simulink model "buoyancy_simulation"  (R2021a)
settings: Solver=ode45  StartTime=0.0  StopTime=180  MaxStep=2.0  RelTol=1e-3
values from neighbouring files (symbols this model uses):
  Cd_bottom = 1    [main_simulation.m]
  Cd_top = 1.28    [main_simulation.m]
  densityProfile = 999    [main_simulation.m]
  depth_CTD = depth_CTD(1:index)    [main_simulation.m]
  g = 9.81    [main_simulation.m]
  integralTreshold = 2    [main_simulation.m]
  Kd = 0.1    [main_simulation.m]
  Ki = 0.001    [main_simulation.m]
  Kp = 0.026    [main_simulation.m]
  offsetSensor = 0    [main_simulation.m]
  sampleTime = 0.5    [main_simulation.m]
  step_depth1 = 10    [main_simulation.m]
  step_depth2 = 5    [main_simulation.m]
  stepTime = 180    [main_simulation.m]
  useCTDprofile = true    [main_simulation.m]
  V_max = V_vehicle + V_outerLid + V_led - V_pistonBlock - V_sensor    [calc_preset_volume.m]
  v_piston_max = 2.44e-3    (= 0.00244)    [main_simulation.m]
undefined symbols (not defined in the file or in its folder): mass, param, rho, sysc
libraries: pid_lib x1
settings Model: Creator=haral  LastModifiedBy=haral
settings SolverCC: ZeroCrossAlgorithm=Adaptive
settings DebuggingCC: IgnoredZcDiagnostic=none

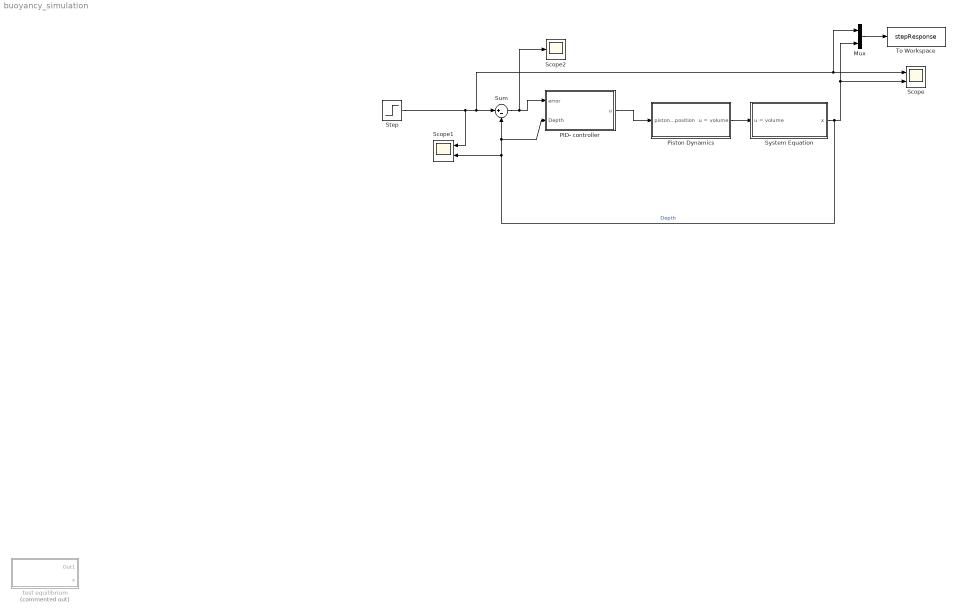
== system buoyancy_simulation ==
  Mux : Mux  Inputs=2
  PID- controller : Subsystem
  Piston Dynamics : Subsystem
  Scope : Scope  NumInputPorts=2
  Scope1 : Scope  NumInputPorts=2
  Scope2 : Scope
  Step : Step  Time=stepTime  Before=step_depth1  After=step_depth2  SampleTime=sampleTime
  Sum : Sum  Inputs=|+-
  System Equation : Subsystem
  To Workspace : ToWorkspace  VariableName=stepResponse  SaveFormat=Structure With Time  SampleTime=-1
  test equilibrium : Subsystem  Commented=on
  wires:
  Step/1 -> Scope1/1, Mux/1, Scope/1, Sum/1
  Sum/1 -> Scope2/1, PID- controller/1(error)
  PID- controller/1(u) -> Piston Dynamics/1(piston position)
  Piston Dynamics/1(u = volume) -> System Equation/1(u = volume)
  System Equation/1(x) -> Sum/2, PID- controller/2(Depth), Scope1/2, Mux/2, Scope/2  "Depth"
  Mux/1 -> To Workspace/1

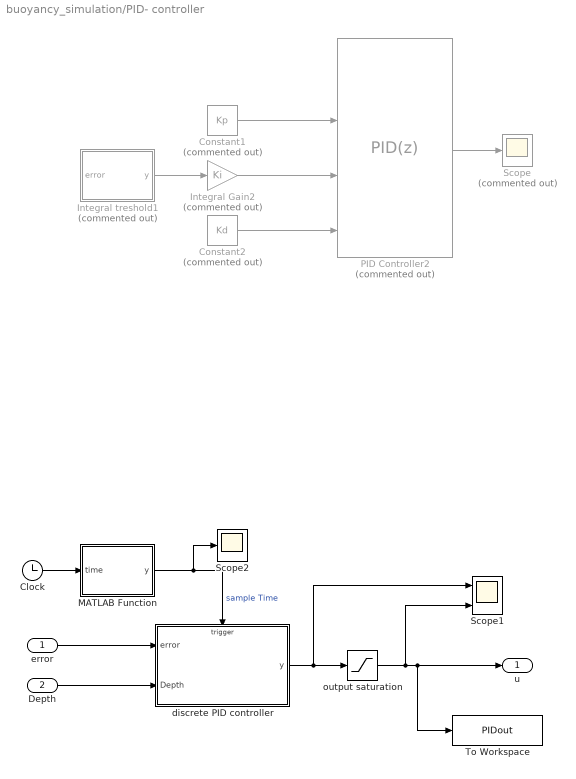
== system buoyancy_simulation/PID- controller ==
  error : Inport
  Depth : Inport  Port=2
  Clock : Clock
  Constant1 : Constant  Commented=on  Value=Kp
  Constant2 : Constant  Commented=on  Value=Kd
  Integral Gain2 : Gain  Commented=on  Gain=Ki
  Integral treshold1 : MATLAB Function  Commented=on  TreatAsAtomicUnit=on
  MATLAB Function : MATLAB Function  TreatAsAtomicUnit=on
  PID Controller2 : pid_lib/PID Controller  Commented=on  Controller=PID  Form=Parallel  TimeDomain=Discrete-time  UseExternalTs=off  SampleTime=0.5  IntegratorMethod=Forward Euler  FilterMethod=Forward Euler  ControllerParametersSource=external  P=Kp  I=Ki  D=Kd  UseFilter=off  N=72.1075704960884  TunerSelectOption=Transfer Function Based (PID Tuner App)  ZeroCross=off  InitialConditionSource=internal  InitialConditionForIntegrator=0  InitialConditionForFilter=0  DifferentiatorICPrevScaledInput=0  ExternalReset=none  TrackingMode=off  Kt=1  LimitOutput=on  SatLimitsSource=internal  UpperSaturationLimit=inf  LowerSaturationLimit=0  LinearizeAsGain=on  AntiWindupMode=none  Kb=1  POutMin=[]  POutMax=[]  IOutMin=[]  IOutMax=[]  DOutMin=[]  DOutMax=[]  NOutMin=[]  NOutMax=[]  SumOutMin=[]  SumOutMax=[]  SaturationOutMin=[]  SaturationOutMax=[]  PParamMin=[]  PParamMax=[]  IParamMin=[]  IParamMax=[]  DParamMin=[]  DParamMax=[]  NParamMin=[]  NParamMax=[]  KbParamMin=[]  KbParamMax=[]  KtParamMin=[]  KtParamMax=[]  KbOutMin=[]  KbOutMax=[]  KtOutMin=[]  KtOutMax=[]  IntegratorOutMin=[]  IntegratorOutMax=[]  FilterOutMin=[]  FilterOutMax=[]  SumI1OutMin=[]  SumI1OutMax=[]  SumI2OutMin=[]  SumI2OutMax=[]  SumI3OutMin=[]  SumI3OutMax=[]  SumI4OutMin=[]  SumI4OutMax=[]  SumDOutMin=[]  SumDOutMax=[]  DifferentiatorOutMin=[]  DifferentiatorOutMax=[]  FilterDiffOutCoefMin=[]  FilterDiffOutCoefMax=[]  ReciprocalOutMin=[]  ReciprocalOutMax=[]  SumDenOutMin=[]  SumDenOutMax=[]  SumNumOutMin=[]  SumNumOutMax=[]  DivideOutMin=[]  DivideOutMax=[]  UdiffTsProdOutMin=[]  UdiffTsProdOutMax=[]  NTsProdOutMin=[]  NTsProdOutMax=[]  UintegralTsProdOutMin=[]  UintegralTsProdOutMax=[]  UngainTsProdOutMin=[]  UngainTsProdOutMax=[]  IntegratorContinuousStateAttributes=''  IntegratorStateMustResolveToSignalObject=off  IntegratorRTWStateStorageClass=Auto  FilterContinuousStateAttributes=''  FilterStateMustResolveToSignalObject=off  FilterRTWStateStorageClass=Auto  ParallelPVariant=ExternalParameters  IdealPVariant=Disabled  IVariant=ExternalParameters  DVariant=ExternalParameters  IntegratorVariant=Discrete  SatVariant=Enabled  AWVariant=Passthrough  PCopyVariant=Disabled  TRVariant=Disabled  FdbkBlocksVariant=Forward  IdealPFdbkVariant=Disabled  SatFdbkVariant=Disabled  DerivativeFilterVariant=Differentiator  NVariant=Passthrough  NCopyVariant=Disabled_SignalSpec  FilterICVariant=InternalICsDifferentiator  IntegratorICVariant=InternalICs  ExternalResetVariant=Disabled  TRSumVariant=Passthrough  SumFdbkVariant=Disabled  SumVariant=Sum_PID  TsampFilterVariant=InternalTs  TsampNgainVariant=Passthrough  TsampIntegralVariant=Passthrough  ExternalSaturationOutDataTypeStr=Inherit: Same as second input
  Scope : Scope  Commented=on
  Scope1 : Scope  NumInputPorts=2
  Scope2 : Scope
  To Workspace : ToWorkspace  VariableName=PIDout  SaveFormat=Structure With Time  SampleTime=-1
  "discrete PID controller " : Subsystem  TreatAsAtomicUnit=on
  output saturation : Saturate  UpperLimit=param.h_piston  LowerLimit=0
  u : Outport
  wires:
  Integral treshold1/1(y) -> Integral Gain2/1
  Constant2/1 -> PID Controller2/4
  Integral Gain2/1 -> PID Controller2/3
  Constant1/1 -> PID Controller2/2
  error/1 -> "discrete PID controller "/1(error)
  "discrete PID controller "/1(y) -> Scope1/1, output saturation/1
  output saturation/1 -> To Workspace/1, u/1, Scope1/2
  MATLAB Function/1(y) -> Scope2/1, "discrete PID controller "/Trigger  "sample Time"
  Clock/1 -> MATLAB Function/1(time)
  PID Controller2/1 -> Scope/1
  Depth/1 -> "discrete PID controller "/2(Depth)

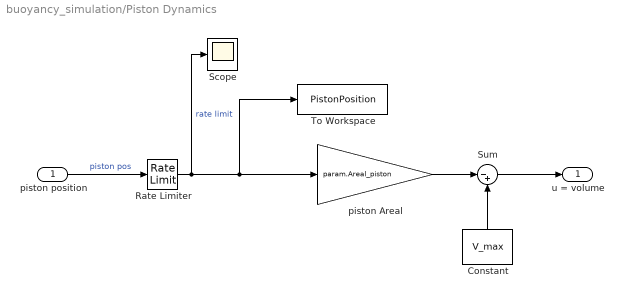
== system buoyancy_simulation/Piston Dynamics ==
  piston position : Inport
  Constant : Constant  Value=V_max
  Rate Limiter : RateLimiter  RisingSlewLimit=v_piston_max  FallingSlewLimit=-v_piston_max  SampleTimeMode=inherited
  Scope : Scope
  Sum : Sum  Inputs=|-+
  To Workspace : ToWorkspace  VariableName=PistonPosition  SaveFormat=Structure With Time  SampleTime=-1
  piston Areal : Gain  Gain=param.Areal_piston
  u = volume : Outport
  wires:
  Rate Limiter/1 -> Scope/1, To Workspace/1, piston Areal/1  "rate limit"
  piston position/1 -> Rate Limiter/1  "piston pos"
  Constant/1 -> Sum/2
  piston Areal/1 -> Sum/1
  Sum/1 -> u = volume/1

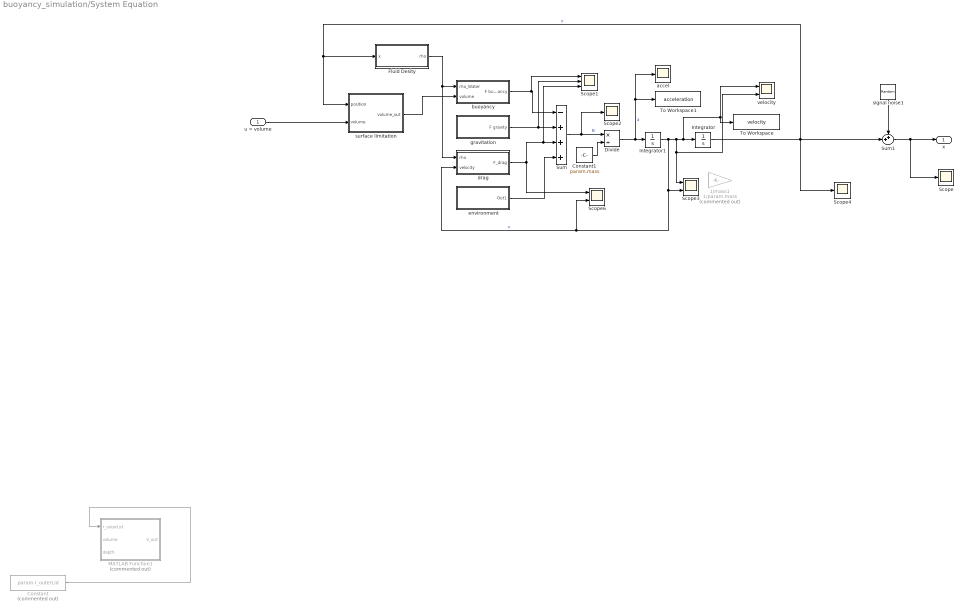
== system buoyancy_simulation/System Equation ==
  u = volume : Inport
  1/mass1 : Gain  Commented=on  Gain=1/param.mass
  Constant : Constant  Commented=on  Value=param.r_outerLid
  Constant1 : Constant  Value=param.mass
  Divide : Product  Inputs=*/
  Fluid Desity : Subsystem
  Integrator : Integrator
  Integrator1 : Integrator
  MATLAB Function1 : MATLAB Function  Commented=on  TreatAsAtomicUnit=on
  Scope : Scope
  Scope1 : Scope  NumInputPorts=3
  Scope2 : Scope
  Scope3 : Scope  NumInputPorts=2
  Scope4 : Scope
  Scope6 : Scope  NumInputPorts=2
  Sum : Sum  Inputs=-+++
  Sum1 : Sum  Inputs=++|
  To Workspace : ToWorkspace  VariableName=velocity  SaveFormat=Structure With Time  SampleTime=-1
  To Workspace1 : ToWorkspace  VariableName=acceleration  SaveFormat=Structure With Time  SampleTime=-1
  accel : Scope
  buoyancy : Subsystem
  drag : Subsystem
  environment : Subsystem
  gravitation : Subsystem
  signal noise1 : RandomNumber  Variance=0.0001  SampleTime=0.5
  surface limitation : MATLAB Function  TreatAsAtomicUnit=on
  velocity : Scope  NumInputPorts=2
  x : Outport
  wires:
  Divide/1 -> accel/1, To Workspace1/1, Integrator1/1  "a"
  Integrator1/1 -> Scope6/2, drag/2(velocity), Scope3/2, velocity/2, Scope3/1, velocity/1, To Workspace/1, Integrator/1  "v"
  buoyancy/1(F buoyancy) -> Scope1/1, Sum/1
  gravitation/1(F gravity) -> Scope1/2, Sum/2
  drag/1(F_drag) -> Scope1/3, Sum/3, Scope6/1
  environment/1(Out1) -> Sum/4
  Fluid Desity/1(rho) -> drag/1(rho), buoyancy/1(rho_Water)
  Sum/1 -> Divide/1, Scope2/1  "N"
  u = volume/1 -> surface limitation/2(volume)
  Integrator/1 -> Sum1/2, surface limitation/1(position), Fluid Desity/1(x), Scope4/1  "x"
  Constant/1 -> MATLAB Function1/1(r_outerLid)
  surface limitation/1(volume_out) -> buoyancy/2(volume)
  signal noise1/1 -> Sum1/1
  Sum1/1 -> Scope/1, x/1
  Constant1/1 -> Divide/2

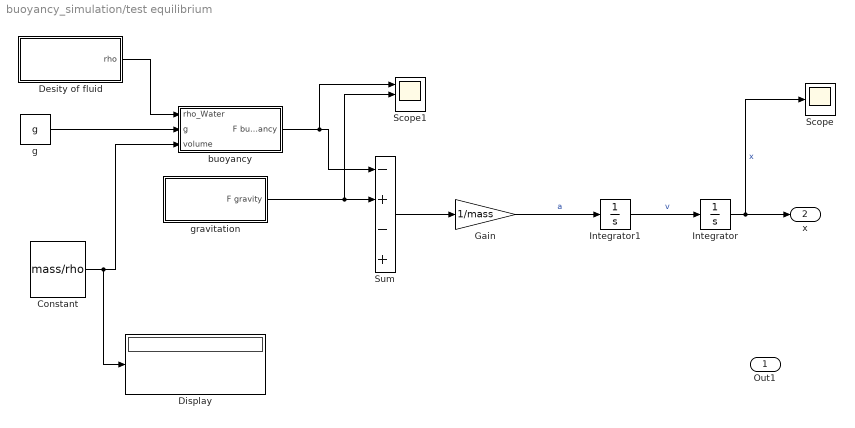
== system buoyancy_simulation/test equilibrium ==
  Constant : Constant  Value=mass/rho
  Desity of fluid : Subsystem
  Display : Display
  Gain : Gain  Gain=1/mass
  Integrator : Integrator
  Integrator1 : Integrator
  Scope : Scope
  Scope1 : Scope  NumInputPorts=3
  Sum : Sum  Inputs=-+-+
  buoyancy : Subsystem
  g : Constant  Value=g
  gravitation : Subsystem
  Out1 : Outport
  x : Outport  Port=2
  wires:
  Constant/1 -> Display/1, buoyancy/3(volume)
  g/1 -> buoyancy/2(g)
  buoyancy/1(F buoyancy) -> Scope1/1, Sum/1
  Gain/1 -> Integrator1/1  "a"
  Integrator/1 -> Scope/1, x/1  "x"
  Desity of fluid/1(rho) -> buoyancy/1(rho_Water)
  Integrator1/1 -> Integrator/1  "v"
  Sum/1 -> Gain/1
  gravitation/1(F gravity) -> Scope1/2, Sum/2

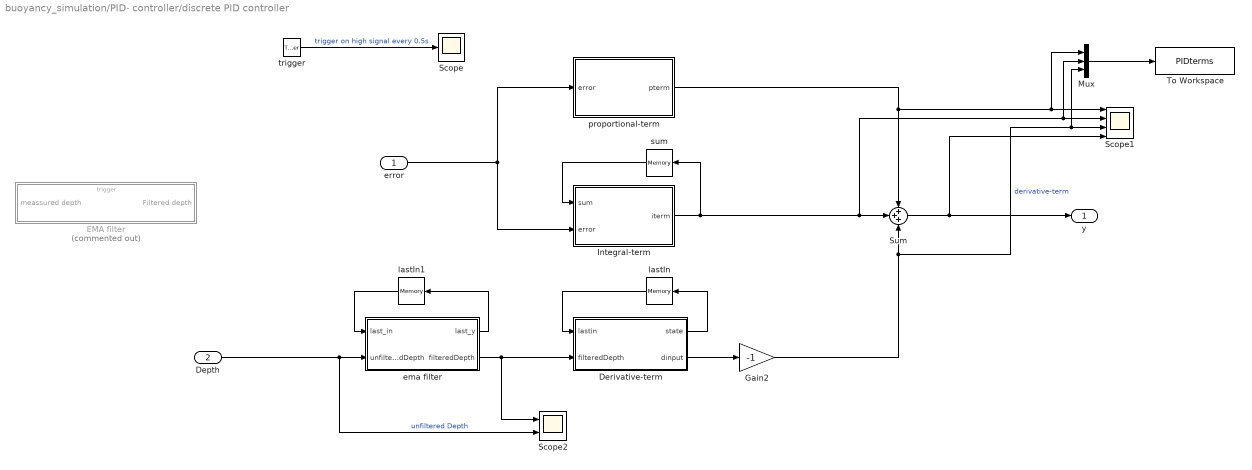
== system buoyancy_simulation/PID- controller/discrete PID controller  ==
  error : Inport
  Depth : Inport  Port=2
  trigger : TriggerPort  VariantControl=(inherit)  ShowOutputPort=on  SampleTimeType=periodic  SampleTime=sampleTime
  Derivative-term : MATLAB Function  TreatAsAtomicUnit=on
  EMA filter : Subsystem  Commented=on
  Gain2 : Gain  Gain=-1
  Integral-term : MATLAB Function  TreatAsAtomicUnit=on
  Mux : Mux  Inputs=3
  Scope : Scope
  Scope1 : Scope  NumInputPorts=4
  Scope2 : Scope  NumInputPorts=2
  Sum : Sum  Inputs=+++
  To Workspace : ToWorkspace  VariableName=PIDterms  SaveFormat=Structure With Time  SampleTime=-1
  ema filter : MATLAB Function  TreatAsAtomicUnit=on
  lastIn : Memory  InheritSampleTime=on
  lastIn1 : Memory  InheritSampleTime=on
  proportional-term : MATLAB Function  TreatAsAtomicUnit=on
  sum : Memory  InheritSampleTime=on
  y : Outport
  wires:
  Integral-term/1(iterm) -> sum/1, Mux/2, Scope1/2, Sum/2
  sum/1 -> Integral-term/1(sum)
  error/1 -> Integral-term/2(error), proportional-term/1(error)
  Depth/1 -> Scope2/2, ema filter/2(unfilteredDepth)  "unfiltered Depth"
  Derivative-term/1(state) -> lastIn/1
  lastIn/1 -> Derivative-term/1(lastin)
  Derivative-term/2(dinput) -> Gain2/1
  Gain2/1 -> Mux/3, Scope1/3, Sum/3  "derivative-term"
  proportional-term/1(pterm) -> Sum/1, Mux/1, Scope1/1
  Sum/1 -> Scope1/4, y/1
  trigger/1 -> Scope/1  "trigger on high signal every 0.5s"
  Mux/1 -> To Workspace/1
  lastIn1/1 -> ema filter/1(last_in)
  ema filter/1(last_y) -> lastIn1/1
  ema filter/2(filteredDepth) -> Scope2/1, Derivative-term/2(filteredDepth)

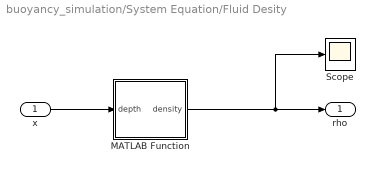
== system buoyancy_simulation/System Equation/Fluid Desity ==
  x : Inport
  MATLAB Function : MATLAB Function  TreatAsAtomicUnit=on
  Scope : Scope
  rho : Outport
  wires:
  MATLAB Function/1(density) -> rho/1, Scope/1
  x/1 -> MATLAB Function/1(depth)

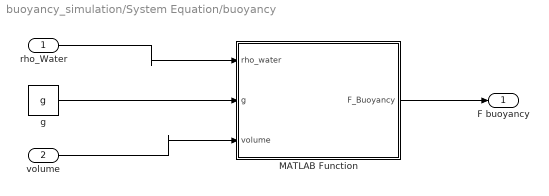
== system buoyancy_simulation/System Equation/buoyancy ==
  rho_Water : Inport
  volume : Inport  Port=2
  MATLAB Function : MATLAB Function  TreatAsAtomicUnit=on
  g : Constant  Value=g
  F buoyancy : Outport
  wires:
  rho_Water/1 -> MATLAB Function/1(rho_water)
  g/1 -> MATLAB Function/2(g)
  volume/1 -> MATLAB Function/3(volume)
  MATLAB Function/1(F_Buoyancy) -> F buoyancy/1

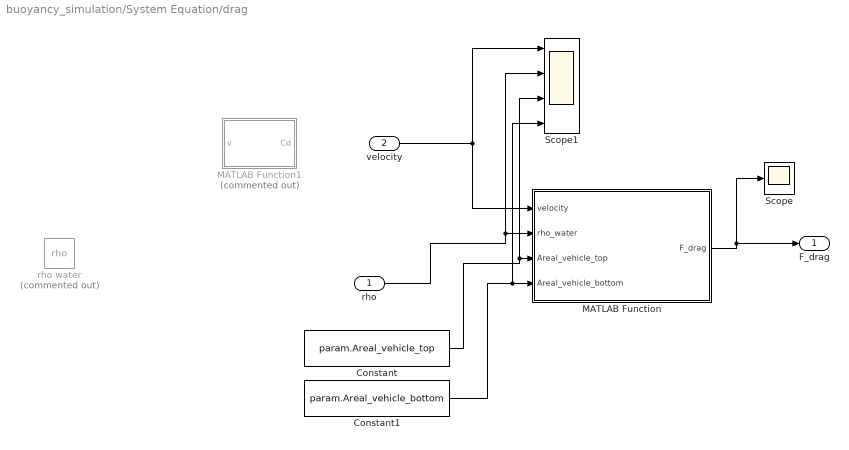
== system buoyancy_simulation/System Equation/drag ==
  rho : Inport
  velocity : Inport  Port=2
  Constant : Constant  Value=param.Areal_vehicle_top
  Constant1 : Constant  Value=param.Areal_vehicle_bottom
  MATLAB Function : MATLAB Function  TreatAsAtomicUnit=on
  MATLAB Function1 : MATLAB Function  Commented=on  TreatAsAtomicUnit=on
  Scope : Scope
  Scope1 : Scope  NumInputPorts=4
  rho water : Constant  Commented=on  Value=rho
  F_drag : Outport
  wires:
  velocity/1 -> Scope1/1, MATLAB Function/1(velocity)
  Constant/1 -> Scope1/3, MATLAB Function/3(Areal_vehicle_top)
  MATLAB Function/1(F_drag) -> Scope/1, F_drag/1
  rho/1 -> Scope1/2, MATLAB Function/2(rho_water)
  Constant1/1 -> Scope1/4, MATLAB Function/4(Areal_vehicle_bottom)

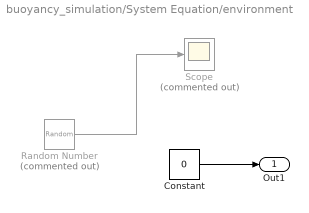
== system buoyancy_simulation/System Equation/environment ==
  Constant : Constant  Value=0
  Random Number : RandomNumber  Commented=on  Variance=0.001  SampleTime=0.1
  Scope : Scope  Commented=on
  Out1 : Outport
  wires:
  Random Number/1 -> Scope/1
  Constant/1 -> Out1/1

== system buoyancy_simulation/System Equation/gravitation ==
  Constant : Constant  Value=param.mass
  Gain : Gain  Gain=g
  F gravity : Outport
  wires:
  Gain/1 -> F gravity/1
  Constant/1 -> Gain/1

== system buoyancy_simulation/test equilibrium/Desity of fluid ==
  Constant : Constant  Value=1000
  rho : Outport
  wires:
  Constant/1 -> rho/1

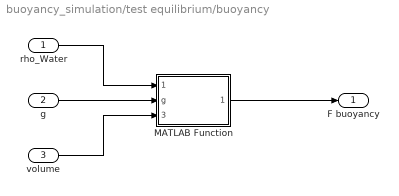
== system buoyancy_simulation/test equilibrium/buoyancy ==
  rho_Water : Inport
  g : Inport  Port=2
  volume : Inport  Port=3
  MATLAB Function : MATLAB Function  TreatAsAtomicUnit=on
  F buoyancy : Outport
  wires:
  rho_Water/1 -> MATLAB Function/1(rho_water)
  g/1 -> MATLAB Function/2(g)
  volume/1 -> MATLAB Function/3(volume)
  MATLAB Function/1(F_Buoyancy) -> F buoyancy/1

== system buoyancy_simulation/test equilibrium/gravitation ==
  Constant : Constant  Value=mass
  Gain : Gain  Gain=g
  F gravity : Outport
  wires:
  Gain/1 -> F gravity/1
  Constant/1 -> Gain/1

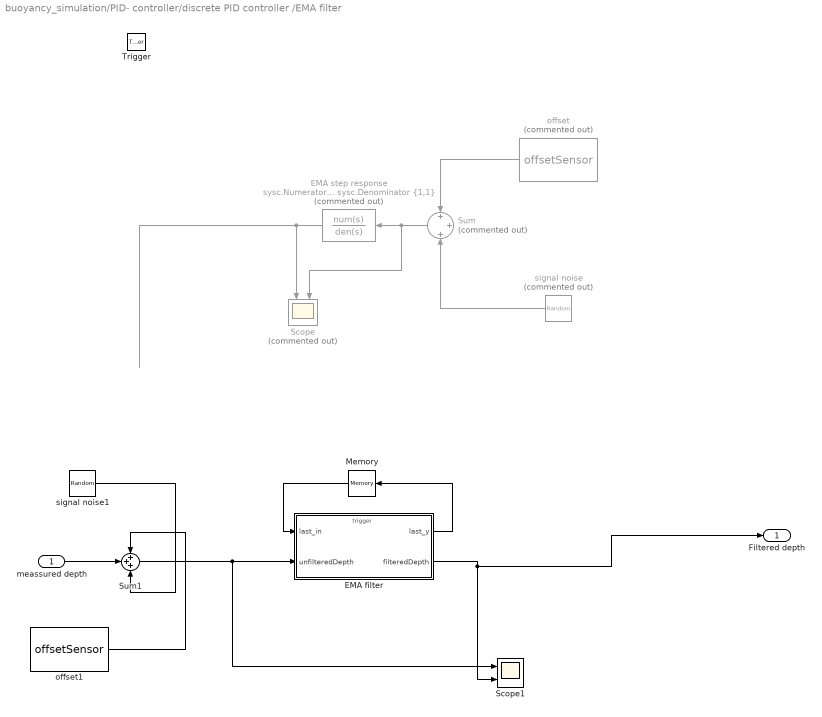
== system buoyancy_simulation/PID- controller/discrete PID controller /EMA filter ==
  meassured depth : Inport
  Trigger : TriggerPort  VariantControl=(inherit)  PortDimensions=1
  EMA filter : MATLAB Function  TreatAsAtomicUnit=on
  EMA step response : TransferFcn  Commented=on  Numerator=sysc.Numerator{1,1}  Denominator=sysc.Denominator {1,1}
  Memory : Memory  InheritSampleTime=on
  Scope : Scope  Commented=on  NumInputPorts=2
  Scope1 : Scope  NumInputPorts=2
  Sum : Sum  Commented=on  Inputs=+|+|+
  Sum1 : Sum  Inputs=+++
  offset : Constant  Commented=on  Value=offsetSensor
  offset1 : Constant  Value=offsetSensor
  signal noise : RandomNumber  Commented=on  Variance=0.0001  SampleTime=0.5
  signal noise1 : RandomNumber  Variance=0.0001  SampleTime=0.5
  Filtered depth : Outport
  wires:
  signal noise/1 -> Sum/3
  ? -> Sum/2
  offset/1 -> Sum/1
  Sum/1 -> Scope/2, EMA step response/1
  EMA step response/1 -> Scope/1
  EMA filter/1(last_y) -> Memory/1
  Memory/1 -> EMA filter/1(last_in)
  EMA filter/2(filteredDepth) -> Scope1/2, Filtered depth/1
  Sum1/1 -> EMA filter/2(unfilteredDepth), Scope1/1
  offset1/1 -> Sum1/1
  signal noise1/1 -> Sum1/3
  meassured depth/1 -> Sum1/2

== matlab function buoyancy_simulation/PID- controller/discrete PID controller /proportional-term ==
  settings: sampleTime=sampleTime
  data: error input; pterm output; Kp parameter
function pterm = fcn(error, Kp)

pterm = Kp*error;
end

== matlab function buoyancy_simulation/System Equation/surface limitation ==
  data: position input; volume input; volume_out output
function volume_out = fcn(position,volume)

if position <= 0
    volume_out = volume - pi*0.025^2*abs(position);
else
    volume_out = volume; 
end

== matlab function buoyancy_simulation/PID- controller/discrete PID controller /ema filter ==
  settings: sampleTime=sampleTime
  data: last_y output; last_in input; unfilteredDepth input; filteredDepth output; alpha parameter
function [last_y,filteredDepth ] = fcn(last_in, unfilteredDepth, alpha)

filteredDepth  =(alpha*unfilteredDepth) + ((1-alpha)*last_in);

%store variable for next calculation
last_y = filteredDepth;
end

== matlab function buoyancy_simulation/System Equation/drag/MATLAB Function1 ==
  data: v input; Cd output
function Cd = fcn(v)
%% not ideal lol
Cd = 0.130/((0.13/2)*(pi/4)*0.13^2*v^2);
end

== matlab function buoyancy_simulation/PID- controller/discrete PID controller /EMA filter/EMA filter ==
  settings: updateMethod=DISCRETE  sampleTime=sampleTime
  data: last_in input; unfilteredDepth input; last_y output; filteredDepth output; alpha parameter
  events: trigger input RISING_EDGE_EVENT
function [last_y,filteredDepth ] = fcn(last_in, unfilteredDepth, alpha)

filteredDepth  =(alpha*unfilteredDepth) + ((1-alpha)*last_in);

%store variable for next calculation
last_y = filteredDepth;
end

== matlab function buoyancy_simulation/System Equation/drag/MATLAB Function ==
  data: velocity input; F_drag output; rho_water input; Areal_vehicle_top input; Areal_vehicle_bottom input; Cd_bottom parameter; Cd_top parameter
function F_drag = fcn(velocity, rho_water, Areal_vehicle_top, Areal_vehicle_bottom, Cd_bottom, Cd_top)

if velocity > 0 % Negative velocity ensure negative drag 
    %floating
    F_drag = - 0.5*Cd_bottom*rho_water*velocity^2*Areal_vehicle_bottom;
    
else % sinking  
    F_drag = 0.5*Cd_top*rho_water*velocity^2*Areal_vehicle_top;
end

== matlab function buoyancy_simulation/System Equation/buoyancy/MATLAB Function ==
  data: rho_water input; F_Buoyancy output; g input; volume input
function F_Buoyancy = fcn(rho_water, g, volume)
%#codegen

F_Buoyancy = rho_water*g*volume;

== matlab function buoyancy_simulation/test equilibrium/buoyancy/MATLAB Function ==
  data: rho_water input; F_Buoyancy output; g input; volume input
function F_Buoyancy = fcn(rho_water, g, volume)
%#codegen

F_Buoyancy = rho_water*g*volume;

== matlab function buoyancy_simulation/System Equation/Fluid Desity/MATLAB Function ==
  data: depth input; density output; densityProfile parameter; depth_CTD parameter; useCTDprofile parameter
function density = fcn(depth, densityProfile, depth_CTD, useCTDprofile)

if useCTDprofile
    if depth <= 0.4
        depth = 0.4;
    end
    index = interp1(depth_CTD, 1:length(depth_CTD), depth, 'nearest'); % find the nearest index of a CTD profile 
    density = densityProfile(index);
else % use constant water density 
    density = densityProfile(1);  
end

end

== matlab function buoyancy_simulation/PID- controller/discrete PID controller /Integral-term ==
  settings: sampleTime=sampleTime
  data: sum input; error input; iterm output; Ki parameter; sampleTime parameter; integralTreshold parameter
function iterm = fcn(sum, error, Ki, sampleTime, integralTreshold)

 if (error < integralTreshold)
    iterm = sum + error*Ki*sampleTime;
    
    %integral wind up
    if iterm > 0.055
        iterm = 0.055;
    elseif iterm < 0
        iterm = 0;
    end
    
 else
     iterm = sum;
end

% function [esum, iterm] = fcn(esum, error, Ki, sampleTime, integralTreshold)
% 
%  if (error < integralTreshold)
%      esum = esum + error;
%     iterm = esum*Ki*sampleTime;
%     
%     %integral wind up
%     if iterm > 0.055
%         iterm = 0.055;
%     elseif iterm < 0
%         iterm = 0;
%     end
%     
%  else
%      iterm = esum;
% end

== matlab function buoyancy_simulation/System Equation/MATLAB Function1 ==
  data: V_out output; r_outerLid input; volume input; depth input
function V_out = fcn( r_outerLid ,volume,  depth)
% Ensure that volume that is floating above the surface dont get buoyancy
% force

if depth <= 0 
    V_out = volume - (depth*pi*r_outerLid^2); % temporaly volume
else
    V_out = volume;
end
end

== matlab function buoyancy_simulation/PID- controller/Integral treshold1 ==
  data: error input; y output; integralTreshold parameter
function y = fcn(error, integralTreshold)

if abs(error) < integralTreshold
    y = 1;
else
    y = 0;
end

end

== matlab function buoyancy_simulation/PID- controller/MATLAB Function ==
  data: time input; y output; sampleTime parameter
function y = fcn(time, sampleTime)

if mod(time, sampleTime) == 0 % to activate every timestep
    y = 1;
else 
    y = 0;
end

== matlab function buoyancy_simulation/PID- controller/discrete PID controller /Derivative-term ==
  settings: sampleTime=sampleTime
  data: state output; lastin input; filteredDepth input; dinput output; sampleTime parameter; Kd parameter
function [state, dinput] = fcn(lastin, filteredDepth, sampleTime, Kd)



%comupute derivative
dinput = ((filteredDepth - lastin)/sampleTime)*Kd; 


% store some variables
state = filteredDepth;
%lastDepth = filteredDepth; %does this work??


disp(sampleTime);
%disp(lastDepth);
